simulink model "Rectifier_1_20kw"  (R2022a)
settings: Solver=VariableStepAuto  StartTime=0.0  StopTime=1.6  RelTol=1e-3
model workspace (MAT data in the model file):
  reset = 0
undefined symbols (not defined in the file): DiscIntNeverNeededParam, lgbt_cap2
libraries: spsSeriesRLCBranchLib x52, spsDiodeLib x14, spsCurrentMeasurementLib x12, slpidlib x10, spsIGBTDiodeLib x8, spsIdealSwitchLib x7, spsVoltageMeasurementLib x7, spsMosfetLib x6, spsLinearTransformerLib x5, spsACVoltageSourceLib x3, spsabctodq0Lib x2, simulink x2
(part 2 of 2)

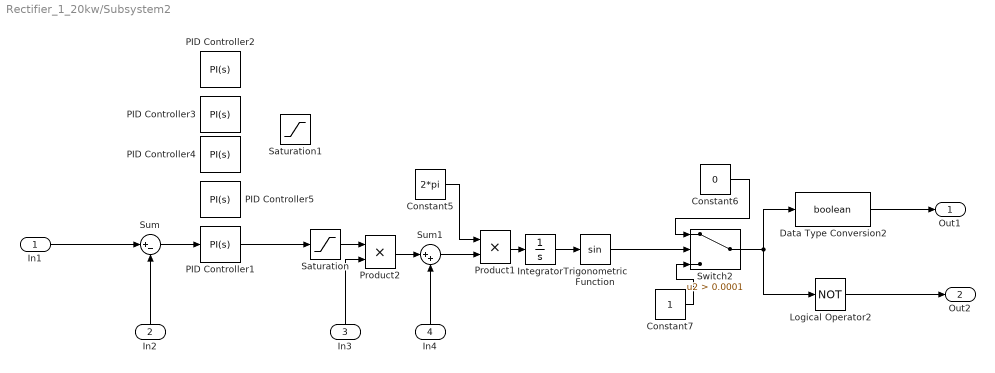
== system Rectifier_1_20kw/Subsystem2 ==
  In1 : Inport
  In2 : Inport  Port=2
  In3 : Inport  Port=3
  In4 : Inport  Port=4
  Constant5 : Constant  Value=2*pi
  Constant6 : Constant  Value=0
  Constant7 : Constant
  Data Type Conversion2 : DataTypeConversion  OutDataTypeStr=boolean  SaturateOnIntegerOverflow=off  RndMeth=Floor
  Integrator : Integrator
  Logical Operator2 : Logic  Operator=NOT  AllPortsSameDT=off  OutDataTypeStr=boolean
  PID Controller1 : slpidlib/PID Controller  Controller=PI  Form=Parallel  TimeDomain=Continuous-time  UseExternalTs=off  SampleTime=-1  IntegratorMethod=Forward Euler  FilterMethod=Forward Euler  ControllerParametersSource=internal  P=P  I=I  UseKiTs=off  D=3  N=100  UseFilter=on  TunerSelectOption=Transfer Function Based (PID Tuner App)  InitialConditionSource=internal  InitialConditionForIntegrator=0  InitialConditionForFilter=0  DifferentiatorICPrevScaledInput=0  ExternalReset=none  TrackingMode=off  Kt=1  LimitOutput=off  SatLimitsSource=internal  UpperSaturationLimit=inf  LowerSaturationLimit=-inf  LinearizeAsGain=on  AntiWindupMode=none  Kb=1  POutMin=[]  POutMax=[]  IOutMin=[]  IOutMax=[]  DOutMin=[]  DOutMax=[]  NOutMin=[]  NOutMax=[]  SumOutMin=[]  SumOutMax=[]  SaturationOutMin=[]  SaturationOutMax=[]  PParamMin=[]  PParamMax=[]  IParamMin=[]  IParamMax=[]  DParamMin=[]  DParamMax=[]  NParamMin=[]  NParamMax=[]  KbParamMin=[]  KbParamMax=[]  KtParamMin=[]  KtParamMax=[]  KbOutMin=[]  KbOutMax=[]  KtOutMin=[]  KtOutMax=[]  IntegratorOutMin=[]  IntegratorOutMax=[]  FilterOutMin=[]  FilterOutMax=[]  SumI1OutMin=[]  SumI1OutMax=[]  SumI2OutMin=[]  SumI2OutMax=[]  SumI3OutMin=[]  SumI3OutMax=[]  SumI4OutMin=[]  SumI4OutMax=[]  SumDOutMin=[]  SumDOutMax=[]  DifferentiatorOutMin=[]  DifferentiatorOutMax=[]  FilterDiffOutCoefMin=[]  FilterDiffOutCoefMax=[]  ReciprocalOutMin=[]  ReciprocalOutMax=[]  SumDenOutMin=[]  SumDenOutMax=[]  SumNumOutMin=[]  SumNumOutMax=[]  DivideOutMin=[]  DivideOutMax=[]  UdiffTsProdOutMin=[]  UdiffTsProdOutMax=[]  NTsProdOutMin=[]  NTsProdOutMax=[]  UintegralTsProdOutMin=[]  UintegralTsProdOutMax=[]  UngainTsProdOutMin=[]  UngainTsProdOutMax=[]  IntegratorContinuousStateAttributes=''  IntegratorStateMustResolveToSignalObject=off  IntegratorRTWStateStorageClass=Auto  FilterContinuousStateAttributes=''  FilterStateMustResolveToSignalObject=off  FilterRTWStateStorageClass=Auto  ParallelPVariant=InternalParameters  IdealPVariant=Disabled  IVariant=InternalParameters  DVariant=Disabled  IntegratorVariant=Continuous  SatVariant=Disabled  AWVariant=Passthrough  PCopyVariant=Disabled  TRVariant=Disabled  FdbkBlocksVariant=Forward  IdealPFdbkVariant=Disabled  SatFdbkVariant=Disabled  DerivativeFilterVariant=Disabled  NVariant=Disabled  NCopyVariant=Disabled_SignalSpec  FilterICVariant=Disabled  IntegratorICVariant=InternalICs  ExternalResetVariant=Disabled  TRSumVariant=Passthrough  SumFdbkVariant=Disabled  SumVariant=Sum_PI  TsampFilterVariant=InternalTs  TsampNgainVariant=Passthrough  TsampIntegralVariant=Passthrough  ExternalSaturationOutDataTypeStr=Inherit: Same as second input  aMode=0
  PID Controller2 : slpidlib/PID Controller  Controller=PI  Form=Parallel  TimeDomain=Continuous-time  UseExternalTs=off  SampleTime=-1  IntegratorMethod=Forward Euler  FilterMethod=Forward Euler  ControllerParametersSource=internal  P=500  I=35000  UseKiTs=off  D=0  N=100  UseFilter=on  TunerSelectOption=Transfer Function Based (PID Tuner App)  InitialConditionSource=internal  InitialConditionForIntegrator=0  InitialConditionForFilter=0  DifferentiatorICPrevScaledInput=0  ExternalReset=none  TrackingMode=off  Kt=1  LimitOutput=off  SatLimitsSource=internal  UpperSaturationLimit=inf  LowerSaturationLimit=-inf  LinearizeAsGain=on  AntiWindupMode=none  Kb=1  POutMin=[]  POutMax=[]  IOutMin=[]  IOutMax=[]  DOutMin=[]  DOutMax=[]  NOutMin=[]  NOutMax=[]  SumOutMin=[]  SumOutMax=[]  SaturationOutMin=[]  SaturationOutMax=[]  PParamMin=[]  PParamMax=[]  IParamMin=[]  IParamMax=[]  DParamMin=[]  DParamMax=[]  NParamMin=[]  NParamMax=[]  KbParamMin=[]  KbParamMax=[]  KtParamMin=[]  KtParamMax=[]  KbOutMin=[]  KbOutMax=[]  KtOutMin=[]  KtOutMax=[]  IntegratorOutMin=[]  IntegratorOutMax=[]  FilterOutMin=[]  FilterOutMax=[]  SumI1OutMin=[]  SumI1OutMax=[]  SumI2OutMin=[]  SumI2OutMax=[]  SumI3OutMin=[]  SumI3OutMax=[]  SumI4OutMin=[]  SumI4OutMax=[]  SumDOutMin=[]  SumDOutMax=[]  DifferentiatorOutMin=[]  DifferentiatorOutMax=[]  FilterDiffOutCoefMin=[]  FilterDiffOutCoefMax=[]  ReciprocalOutMin=[]  ReciprocalOutMax=[]  SumDenOutMin=[]  SumDenOutMax=[]  SumNumOutMin=[]  SumNumOutMax=[]  DivideOutMin=[]  DivideOutMax=[]  UdiffTsProdOutMin=[]  UdiffTsProdOutMax=[]  NTsProdOutMin=[]  NTsProdOutMax=[]  UintegralTsProdOutMin=[]  UintegralTsProdOutMax=[]  UngainTsProdOutMin=[]  UngainTsProdOutMax=[]  IntegratorContinuousStateAttributes=''  IntegratorStateMustResolveToSignalObject=off  IntegratorRTWStateStorageClass=Auto  FilterContinuousStateAttributes=''  FilterStateMustResolveToSignalObject=off  FilterRTWStateStorageClass=Auto  ParallelPVariant=InternalParameters  IdealPVariant=Disabled  IVariant=InternalParameters  DVariant=Disabled  IntegratorVariant=Continuous  SatVariant=Disabled  AWVariant=Passthrough  PCopyVariant=Disabled  TRVariant=Disabled  FdbkBlocksVariant=Forward  IdealPFdbkVariant=Disabled  SatFdbkVariant=Disabled  DerivativeFilterVariant=Disabled  NVariant=Disabled  NCopyVariant=Disabled_SignalSpec  FilterICVariant=Disabled  IntegratorICVariant=InternalICs  ExternalResetVariant=Disabled  TRSumVariant=Passthrough  SumFdbkVariant=Disabled  SumVariant=Sum_PI  TsampFilterVariant=InternalTs  TsampNgainVariant=Passthrough  TsampIntegralVariant=Passthrough  ExternalSaturationOutDataTypeStr=Inherit: Same as second input  aMode=0
  PID Controller3 : slpidlib/PID Controller  Controller=PI  Form=Parallel  TimeDomain=Continuous-time  UseExternalTs=off  SampleTime=-1  IntegratorMethod=Forward Euler  FilterMethod=Forward Euler  ControllerParametersSource=internal  P=1400  I=45000  UseKiTs=off  D=0  N=100  UseFilter=on  TunerSelectOption=Transfer Function Based (PID Tuner App)  InitialConditionSource=internal  InitialConditionForIntegrator=0  InitialConditionForFilter=0  DifferentiatorICPrevScaledInput=0  ExternalReset=none  TrackingMode=off  Kt=1  LimitOutput=off  SatLimitsSource=internal  UpperSaturationLimit=inf  LowerSaturationLimit=-inf  LinearizeAsGain=on  AntiWindupMode=none  Kb=1  POutMin=[]  POutMax=[]  IOutMin=[]  IOutMax=[]  DOutMin=[]  DOutMax=[]  NOutMin=[]  NOutMax=[]  SumOutMin=[]  SumOutMax=[]  SaturationOutMin=[]  SaturationOutMax=[]  PParamMin=[]  PParamMax=[]  IParamMin=[]  IParamMax=[]  DParamMin=[]  DParamMax=[]  NParamMin=[]  NParamMax=[]  KbParamMin=[]  KbParamMax=[]  KtParamMin=[]  KtParamMax=[]  KbOutMin=[]  KbOutMax=[]  KtOutMin=[]  KtOutMax=[]  IntegratorOutMin=[]  IntegratorOutMax=[]  FilterOutMin=[]  FilterOutMax=[]  SumI1OutMin=[]  SumI1OutMax=[]  SumI2OutMin=[]  SumI2OutMax=[]  SumI3OutMin=[]  SumI3OutMax=[]  SumI4OutMin=[]  SumI4OutMax=[]  SumDOutMin=[]  SumDOutMax=[]  DifferentiatorOutMin=[]  DifferentiatorOutMax=[]  FilterDiffOutCoefMin=[]  FilterDiffOutCoefMax=[]  ReciprocalOutMin=[]  ReciprocalOutMax=[]  SumDenOutMin=[]  SumDenOutMax=[]  SumNumOutMin=[]  SumNumOutMax=[]  DivideOutMin=[]  DivideOutMax=[]  UdiffTsProdOutMin=[]  UdiffTsProdOutMax=[]  NTsProdOutMin=[]  NTsProdOutMax=[]  UintegralTsProdOutMin=[]  UintegralTsProdOutMax=[]  UngainTsProdOutMin=[]  UngainTsProdOutMax=[]  IntegratorContinuousStateAttributes=''  IntegratorStateMustResolveToSignalObject=off  IntegratorRTWStateStorageClass=Auto  FilterContinuousStateAttributes=''  FilterStateMustResolveToSignalObject=off  FilterRTWStateStorageClass=Auto  ParallelPVariant=InternalParameters  IdealPVariant=Disabled  IVariant=InternalParameters  DVariant=Disabled  IntegratorVariant=Continuous  SatVariant=Disabled  AWVariant=Passthrough  PCopyVariant=Disabled  TRVariant=Disabled  FdbkBlocksVariant=Forward  IdealPFdbkVariant=Disabled  SatFdbkVariant=Disabled  DerivativeFilterVariant=Disabled  NVariant=Disabled  NCopyVariant=Disabled_SignalSpec  FilterICVariant=Disabled  IntegratorICVariant=InternalICs  ExternalResetVariant=Disabled  TRSumVariant=Passthrough  SumFdbkVariant=Disabled  SumVariant=Sum_PI  TsampFilterVariant=InternalTs  TsampNgainVariant=Passthrough  TsampIntegralVariant=Passthrough  ExternalSaturationOutDataTypeStr=Inherit: Same as second input  aMode=0
  PID Controller4 : slpidlib/PID Controller  Controller=PI  Form=Parallel  TimeDomain=Continuous-time  UseExternalTs=off  SampleTime=-1  IntegratorMethod=Forward Euler  FilterMethod=Forward Euler  ControllerParametersSource=internal  P=5000  I=20000  UseKiTs=off  D=0  N=100  UseFilter=on  TunerSelectOption=Transfer Function Based (PID Tuner App)  InitialConditionSource=internal  InitialConditionForIntegrator=0  InitialConditionForFilter=0  DifferentiatorICPrevScaledInput=0  ExternalReset=none  TrackingMode=off  Kt=1  LimitOutput=off  SatLimitsSource=internal  UpperSaturationLimit=inf  LowerSaturationLimit=-inf  LinearizeAsGain=on  AntiWindupMode=none  Kb=1  POutMin=[]  POutMax=[]  IOutMin=[]  IOutMax=[]  DOutMin=[]  DOutMax=[]  NOutMin=[]  NOutMax=[]  SumOutMin=[]  SumOutMax=[]  SaturationOutMin=[]  SaturationOutMax=[]  PParamMin=[]  PParamMax=[]  IParamMin=[]  IParamMax=[]  DParamMin=[]  DParamMax=[]  NParamMin=[]  NParamMax=[]  KbParamMin=[]  KbParamMax=[]  KtParamMin=[]  KtParamMax=[]  KbOutMin=[]  KbOutMax=[]  KtOutMin=[]  KtOutMax=[]  IntegratorOutMin=[]  IntegratorOutMax=[]  FilterOutMin=[]  FilterOutMax=[]  SumI1OutMin=[]  SumI1OutMax=[]  SumI2OutMin=[]  SumI2OutMax=[]  SumI3OutMin=[]  SumI3OutMax=[]  SumI4OutMin=[]  SumI4OutMax=[]  SumDOutMin=[]  SumDOutMax=[]  DifferentiatorOutMin=[]  DifferentiatorOutMax=[]  FilterDiffOutCoefMin=[]  FilterDiffOutCoefMax=[]  ReciprocalOutMin=[]  ReciprocalOutMax=[]  SumDenOutMin=[]  SumDenOutMax=[]  SumNumOutMin=[]  SumNumOutMax=[]  DivideOutMin=[]  DivideOutMax=[]  UdiffTsProdOutMin=[]  UdiffTsProdOutMax=[]  NTsProdOutMin=[]  NTsProdOutMax=[]  UintegralTsProdOutMin=[]  UintegralTsProdOutMax=[]  UngainTsProdOutMin=[]  UngainTsProdOutMax=[]  IntegratorContinuousStateAttributes=''  IntegratorStateMustResolveToSignalObject=off  IntegratorRTWStateStorageClass=Auto  FilterContinuousStateAttributes=''  FilterStateMustResolveToSignalObject=off  FilterRTWStateStorageClass=Auto  ParallelPVariant=InternalParameters  IdealPVariant=Disabled  IVariant=InternalParameters  DVariant=Disabled  IntegratorVariant=Continuous  SatVariant=Disabled  AWVariant=Passthrough  PCopyVariant=Disabled  TRVariant=Disabled  FdbkBlocksVariant=Forward  IdealPFdbkVariant=Disabled  SatFdbkVariant=Disabled  DerivativeFilterVariant=Disabled  NVariant=Disabled  NCopyVariant=Disabled_SignalSpec  FilterICVariant=Disabled  IntegratorICVariant=InternalICs  ExternalResetVariant=Disabled  TRSumVariant=Passthrough  SumFdbkVariant=Disabled  SumVariant=Sum_PI  TsampFilterVariant=InternalTs  TsampNgainVariant=Passthrough  TsampIntegralVariant=Passthrough  ExternalSaturationOutDataTypeStr=Inherit: Same as second input  aMode=0
  PID Controller5 : slpidlib/PID Controller  Controller=PI  Form=Parallel  TimeDomain=Continuous-time  UseExternalTs=off  SampleTime=-1  IntegratorMethod=Forward Euler  FilterMethod=Forward Euler  ControllerParametersSource=internal  P=3150  I=13200  UseKiTs=off  D=3  N=100  UseFilter=on  TunerSelectOption=Transfer Function Based (PID Tuner App)  InitialConditionSource=internal  InitialConditionForIntegrator=0  InitialConditionForFilter=0  DifferentiatorICPrevScaledInput=0  ExternalReset=none  TrackingMode=off  Kt=1  LimitOutput=off  SatLimitsSource=internal  UpperSaturationLimit=inf  LowerSaturationLimit=-inf  LinearizeAsGain=on  AntiWindupMode=none  Kb=1  POutMin=[]  POutMax=[]  IOutMin=[]  IOutMax=[]  DOutMin=[]  DOutMax=[]  NOutMin=[]  NOutMax=[]  SumOutMin=[]  SumOutMax=[]  SaturationOutMin=[]  SaturationOutMax=[]  PParamMin=[]  PParamMax=[]  IParamMin=[]  IParamMax=[]  DParamMin=[]  DParamMax=[]  NParamMin=[]  NParamMax=[]  KbParamMin=[]  KbParamMax=[]  KtParamMin=[]  KtParamMax=[]  KbOutMin=[]  KbOutMax=[]  KtOutMin=[]  KtOutMax=[]  IntegratorOutMin=[]  IntegratorOutMax=[]  FilterOutMin=[]  FilterOutMax=[]  SumI1OutMin=[]  SumI1OutMax=[]  SumI2OutMin=[]  SumI2OutMax=[]  SumI3OutMin=[]  SumI3OutMax=[]  SumI4OutMin=[]  SumI4OutMax=[]  SumDOutMin=[]  SumDOutMax=[]  DifferentiatorOutMin=[]  DifferentiatorOutMax=[]  FilterDiffOutCoefMin=[]  FilterDiffOutCoefMax=[]  ReciprocalOutMin=[]  ReciprocalOutMax=[]  SumDenOutMin=[]  SumDenOutMax=[]  SumNumOutMin=[]  SumNumOutMax=[]  DivideOutMin=[]  DivideOutMax=[]  UdiffTsProdOutMin=[]  UdiffTsProdOutMax=[]  NTsProdOutMin=[]  NTsProdOutMax=[]  UintegralTsProdOutMin=[]  UintegralTsProdOutMax=[]  UngainTsProdOutMin=[]  UngainTsProdOutMax=[]  IntegratorContinuousStateAttributes=''  IntegratorStateMustResolveToSignalObject=off  IntegratorRTWStateStorageClass=Auto  FilterContinuousStateAttributes=''  FilterStateMustResolveToSignalObject=off  FilterRTWStateStorageClass=Auto  ParallelPVariant=InternalParameters  IdealPVariant=Disabled  IVariant=InternalParameters  DVariant=Disabled  IntegratorVariant=Continuous  SatVariant=Disabled  AWVariant=Passthrough  PCopyVariant=Disabled  TRVariant=Disabled  FdbkBlocksVariant=Forward  IdealPFdbkVariant=Disabled  SatFdbkVariant=Disabled  DerivativeFilterVariant=Disabled  NVariant=Disabled  NCopyVariant=Disabled_SignalSpec  FilterICVariant=Disabled  IntegratorICVariant=InternalICs  ExternalResetVariant=Disabled  TRSumVariant=Passthrough  SumFdbkVariant=Disabled  SumVariant=Sum_PI  TsampFilterVariant=InternalTs  TsampNgainVariant=Passthrough  TsampIntegralVariant=Passthrough  ExternalSaturationOutDataTypeStr=Inherit: Same as second input  aMode=0
  Product1 : Product
  Product2 : Product
  Saturation : Saturate  UpperLimit=3750  LowerLimit=-3600
  Saturation1 : Saturate  UpperLimit=6000  LowerLimit=-3000
  Sum : Sum  Inputs=|+-
  Sum1 : Sum  Inputs=|++
  Switch2 : Switch  Criteria=u2 > Threshold  Threshold=0.0001  ZeroCross=off  SaturateOnIntegerOverflow=off  InputSameDT=off
  Trigonometric Function : Trigonometry
  Out1 : Outport
  Out2 : Outport  Port=2
  wires:
  PID Controller1/1 -> Saturation/1
  Integrator/1 -> Trigonometric Function/1
  Product1/1 -> Integrator/1
  Constant7/1 -> Switch2/3
  Logical Operator2/1 -> Out2/1
  Data Type Conversion2/1 -> Out1/1
  In1/1 -> Sum/1
  Sum/1 -> PID Controller1/1
  Trigonometric Function/1 -> Switch2/2
  Switch2/1 -> Data Type Conversion2/1, Logical Operator2/1
  Constant6/1 -> Switch2/1
  In2/1 -> Sum/2
  Constant5/1 -> Product1/1
  In3/1 -> Product2/2
  Saturation/1 -> Product2/1
  Product2/1 -> Sum1/1
  Sum1/1 -> Product1/2
  In4/1 -> Sum1/2

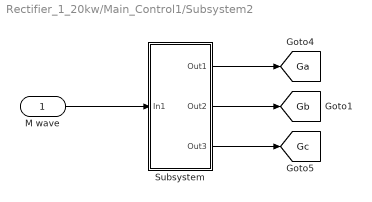
== system Rectifier_1_20kw/Main_Control1/Subsystem2 ==
  M wave : Inport
  Subsystem : Subsystem
  tag scope: Ga=global, Gb=global, Gc=global
  wires:
  M wave/1 -> Subsystem/1(In1)
  Subsystem/1(Out1) -> [Ga]
  Subsystem/2(Out2) -> [Gb]
  Subsystem/3(Out3) -> [Gc]

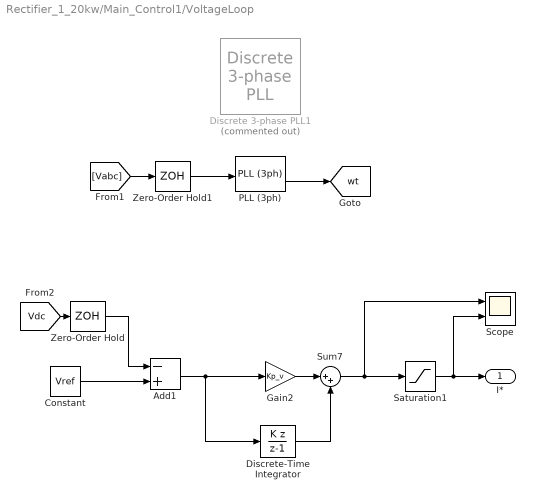
== system Rectifier_1_20kw/Main_Control1/VoltageLoop ==
  Add1 : Sum  Inputs=-+
  Constant : Constant  Value=Vref
  Discrete 3-phase PLL1 : powerlib_extras/Discrete  Control Blocks/Discrete 3-phase PLL  Commented=on  Fmin=45  Par_Init=[0 50]  ParK=[ 180 3200 1 ]  Ts=50e-6  AGC=off
      settings: SourceProductBaseCode=PS
  Discrete-Time Integrator : DiscreteIntegrator  IntegratorMethod=Accumulation: Backward Euler  gainval=Ki_v  SampleTime=1/Fs/2  ICPrevOutput=DiscIntNeverNeededParam  ICPrevScaledInput=DiscIntNeverNeededParam
  Gain2 : Gain  Gain=Kp_v
  PLL (3ph) : spsPLL3phLib/PLL (3ph)  Fmin=45  Par_Init=[0, 60]  ParK=[180, 3200, 1]  TcD=1e-4  MaxRateChangeFreq=12  FilterCutOffFreq=25  Ts=0  AGC=on
  Saturation1 : Saturate  UpperLimit=limit1  LowerLimit=-limit1  SampleTime=1/Fs/2
  Scope : Scope  NumInputPorts=2
  Sum7 : Sum  Inputs=|++
  Zero-Order Hold : ZeroOrderHold  SampleTime=1/Fs/2
  Zero-Order Hold1 : ZeroOrderHold  SampleTime=1/Fs/2
  I* : Outport
  tag scope: wt=global
  wires:
  [Vdc] -> Zero-Order Hold/1
  Zero-Order Hold/1 -> Add1/1
  Constant/1 -> Add1/2
  Saturation1/1 -> I*/1, Scope/2
  Add1/1 -> Discrete-Time Integrator/1, Gain2/1
  Gain2/1 -> Sum7/1
  Discrete-Time Integrator/1 -> Sum7/2
  Sum7/1 -> Scope/1, Saturation1/1
  [Vabc] -> Zero-Order Hold1/1
  Zero-Order Hold1/1 -> PLL (3ph)/1
  PLL (3ph)/2 -> [wt]

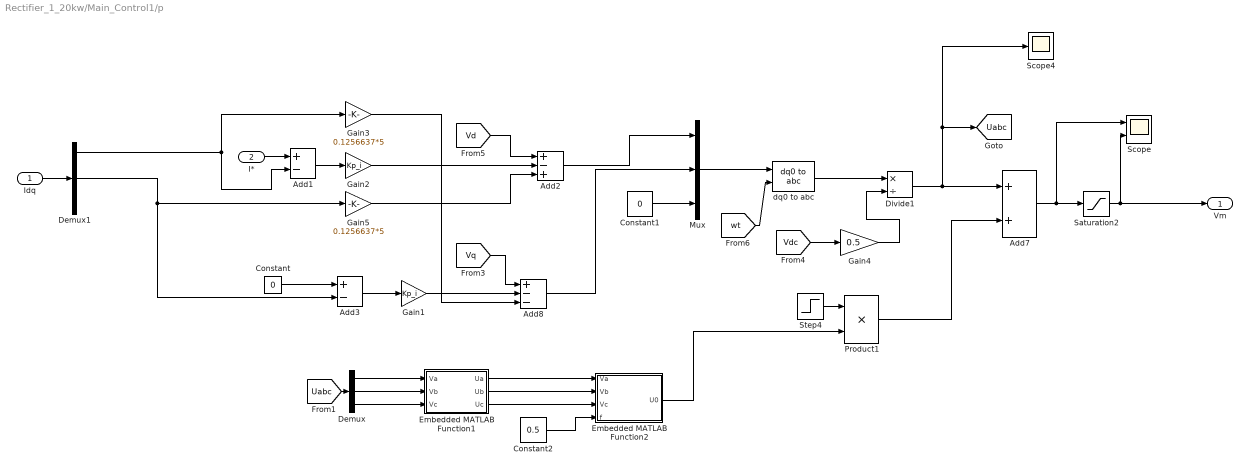
== system Rectifier_1_20kw/Main_Control1/p ==
  Idq : Inport
  I* : Inport  Port=2
  Add1 : Sum  Inputs=+-
  Add2 : Sum  Inputs=+-+
  Add3 : Sum  Inputs=+-
  Add7 : Sum
  Add8 : Sum  Inputs=+--
  Constant : Constant  Value=0
  Constant1 : Constant  Value=0
  Constant2 : Constant  Value=0.5
  Demux : Demux  Outputs=3
  Demux1 : Demux  Outputs=3
  Divide1 : Product  Inputs=*/
  Embedded MATLAB Function1 : MATLAB Function  TreatAsAtomicUnit=on
  Embedded MATLAB Function2 : MATLAB Function  TreatAsAtomicUnit=on
  Gain1 : Gain  Gain=Kp_i  SampleTime=1/Fs/2
  Gain2 : Gain  Gain=Kp_i  SampleTime=1/Fs/2
  Gain3 : Gain  Gain=0.1256637*5  SampleTime=1/Fs/2
  Gain4 : Gain  Gain=0.5  SampleTime=1/Fs/2
  Gain5 : Gain  Gain=0.1256637*5  SampleTime=1/Fs/2
  Mux : Mux  Inputs=3
  Product1 : Product
  Saturation2 : Saturate  UpperLimit=1  LowerLimit=-1  SampleTime=1/Fs/2
  Scope : Scope  NumInputPorts=2
  Scope4 : Scope
  Step4 : Step  Time=0.2  SampleTime=0
  dq0 to abc : spsdq0toabcLib/dq0 to abc  Alignment=90 degrees behind phase A axis
  Vm : Outport
  tag scope: Uabc=global
  wires:
  Idq/1 -> Demux1/1
  Gain3/1 -> Add8/3
  Add3/1 -> Gain1/1
  Add1/1 -> Gain2/1
  [Vq] -> Add8/1
  Gain5/1 -> Add2/3
  [Vd] -> Add2/1
  Add8/1 -> Mux/2
  Mux/1 -> dq0 to abc/1
  Constant1/1 -> Mux/3
  Add2/1 -> Mux/1
  [Vdc] -> Gain4/1
  Saturation2/1 -> Vm/1, Scope/2
  Add7/1 -> Scope/1, Saturation2/1
  Demux1/2 -> Add3/2, Gain5/1
  Demux1/1 -> Gain3/1, Add1/2
  Gain2/1 -> Add2/2
  Gain1/1 -> Add8/2
  Gain4/1 -> Divide1/2
  Divide1/1 -> [Uabc], Scope4/1, Add7/1
  Step4/1 -> Product1/1
  Embedded MATLAB Function2/1(U0) -> Product1/2
  [Uabc] -> Demux/1
  Embedded MATLAB Function1/2(Ub) -> Embedded MATLAB Function2/2(Vb)
  Demux/3 -> Embedded MATLAB Function1/3(Vc)
  Demux/2 -> Embedded MATLAB Function1/2(Vb)
  Demux/1 -> Embedded MATLAB Function1/1(Va)
  Embedded MATLAB Function1/1(Ua) -> Embedded MATLAB Function2/1(Va)
  Embedded MATLAB Function1/3(Uc) -> Embedded MATLAB Function2/3(Vc)
  Constant2/1 -> Embedded MATLAB Function2/4(f)
  [wt] -> dq0 to abc/2
  dq0 to abc/1 -> Divide1/1
  Constant/1 -> Add3/1
  I*/1 -> Add1/1
  Product1/1 -> Add7/2

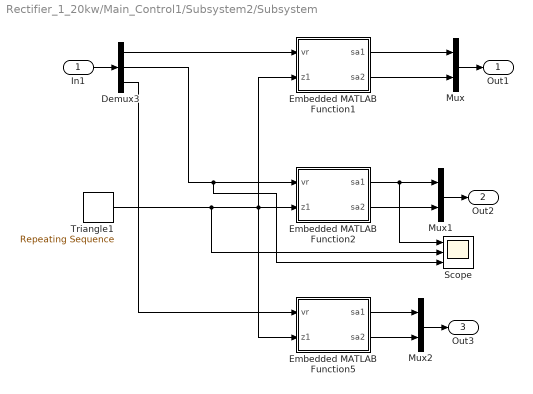
== system Rectifier_1_20kw/Main_Control1/Subsystem2/Subsystem ==
  In1 : Inport
  Demux3 : Demux  Outputs=3
  Embedded MATLAB Function1 : MATLAB Function  TreatAsAtomicUnit=on
  Embedded MATLAB Function2 : MATLAB Function  TreatAsAtomicUnit=on
  Embedded MATLAB Function5 : MATLAB Function  TreatAsAtomicUnit=on
  Mux : Mux  Inputs=2
  Mux1 : Mux  Inputs=2
  Mux2 : Mux  Inputs=2
  Scope : Scope  NumInputPorts=3
  Triangle1 : simulink/Sources/Repeating Sequence  rep_seq_t=[0 0.5/Fs 1/Fs]  rep_seq_y=[0 1 0]
  Out1 : Outport
  Out2 : Outport  Port=2
  Out3 : Outport  Port=3
  wires:
  Triangle1/1 -> Scope/2, Embedded MATLAB Function1/2(z1), Embedded MATLAB Function2/2(z1), Embedded MATLAB Function5/2(z1)
  Demux3/1 -> Embedded MATLAB Function1/1(vr)
  Demux3/2 -> Scope/3, Embedded MATLAB Function2/1(vr)
  Demux3/3 -> Embedded MATLAB Function5/1(vr)
  Embedded MATLAB Function1/1(sa1) -> Mux/1
  Embedded MATLAB Function1/2(sa2) -> Mux/2
  Embedded MATLAB Function2/1(sa1) -> Scope/1, Mux1/1
  Embedded MATLAB Function2/2(sa2) -> Mux1/2
  Embedded MATLAB Function5/1(sa1) -> Mux2/1
  Embedded MATLAB Function5/2(sa2) -> Mux2/2
  In1/1 -> Demux3/1
  Mux/1 -> Out1/1
  Mux1/1 -> Out2/1
  Mux2/1 -> Out3/1

== matlab function Rectifier_1_20kw/Main_Control1/Subsystem2/Subsystem/Embedded MATLAB Function1 ==
  data: vr input; sa1 output; z1 input; sa2 output
function [sa1,sa2] = PDWM(vr,z1)
% This block supports the Embedded MATLAB subset.
% See the help menu for details.
% Initial for persistent variable
if(vr>0) %zhengbanzhouqi 
    if(vr>z1)
        sa1=0;sa2=1;
    else
        sa1=1;sa2=1;
    end
else     %fubanzhouqi
    vr=vr+1;
    if(vr>z1)
        sa1=1;sa2=1;
    else
        sa1=1;sa2=0;
    end
end

== matlab function Rectifier_1_20kw/Main_Control1/Subsystem2/Subsystem/Embedded MATLAB Function2 ==
  data: vr input; sa1 output; z1 input; sa2 output
function [sa1,sa2] = PDWM(vr,z1)
% This block supports the Embedded MATLAB subset.
% See the help menu for details.
% Initial for persistent variable
if(vr>0) %zhengbanzhouqi 
    if(vr>z1)
        sa1=0;sa2=1;
    else
        sa1=1;sa2=1;
    end
else     %fubanzhouqi
    vr=vr+1;
    if(vr>z1)
        sa1=1;sa2=1;
    else
        sa1=1;sa2=0;
    end
end

== matlab function Rectifier_1_20kw/Main_Control1/Subsystem2/Subsystem/Embedded MATLAB Function5 ==
  data: vr input; sa1 output; z1 input; sa2 output
function [sa1,sa2] = PDWM(vr,z1)
% This block supports the Embedded MATLAB subset.
% See the help menu for details.
% Initial for persistent variable
if(vr>0) %zhengbanzhouqi 
    if(vr>z1)
        sa1=0;sa2=1;
    else
        sa1=1;sa2=1;
    end
else     %fubanzhouqi
    vr=vr+1;
    if(vr>z1)
        sa1=1;sa2=1;
    else
        sa1=1;sa2=0;
    end
end

== matlab function Rectifier_1_20kw/Main_Control1/p/Embedded MATLAB Function1 ==
  data: Va input; Ua output; Vb input; Ub output; Vc input; Uc output
function [Ua,Ub,Uc] = fcn(Va,Vb,Vc)

if Va>=0;
    Ua=Va;
else
    Ua=Va+1;
end
if Vb>=0;
    Ub=Vb;
else
    Ub=Vb+1;
end
if Vc>=0;
    Uc=Vc;
else
    Uc=Vc+1;
end

== matlab function Rectifier_1_20kw/Main_Control1/p/Embedded MATLAB Function2 ==
  data: Va input; U0 output; Vb input; Vc input; f input
function U0  = fcn(Va,Vb,Vc,f)

Vmax=Va;         
Vmin=Va;
if Va>=Vb
    Vmin=Vb;
else
    Vmax=Vb;
end
if Vc>=Vmax
    Vmax=Vc;
else 
end
if Vc<=Vmin
    Vmin=Vc;
else
end
U0=f*(1-Vmax+Vmin)-Vmin;
end
